simulink model "FlshbcontrolHybridefinal"  (R2020a)
settings: Solver=VariableStepAuto  StartTime=0.0  StopTime=400  RelTol=1e-3
values from neighbouring files (symbols this model uses):
  Acure = Afb    [Initiate.m]
  Afb = [1.9325, 1 ... (first row only)    [Initiate.m]
  Anf = 0.9855    [Initiate.m]
  Anom = 0.9989    [Initiate.m]
  Bcure = 2/7*Bfb    [Initiate.m]
  Bfb = [16.4988 ... (first row only)    [Initiate.m]
  Bnf = -1.5360/4    (= -0.384)    [Initiate.m]
  Bnom = -1.4118e-05    [Initiate.m]
  Ccure = Cfb    [Initiate.m]
  Cfb = [1, 0]    [Initiate.m]
  Cnf = 1    [Initiate.m]
  Cnom = 1    [Initiate.m]
  Dtmax = 2    [Initiate.m]
  dTulim = 3.8    [Initiate.m]
  eta_switch = 0.05    [Initiate.m]
  F = [107.404393816111,9.22073025292975]    [Initiate.m]
  Re2 = [42000000 42000000 42000000 42000000 42000000 42000000 42000000 42000000 42000000 42000000 42000000 42000000 ... (2604 elements, 1302x2)]    [data.mat]
  TC2 = [50.3264 50.3264 50.3264 50.3264 50.3264 50.4703 50.4703 50.3264 50.4703 50.1825 50.4703 50.4703 ... (43248 elements, 10812x4)]    [data.mat]
  Tref = 55*ones(size(t))    [Initiate.m]
  ts = 1/fs    (= 0.02)    [Initiate.m]
libraries: simulink x4, dspsrcs4 x3
settings Model: Creator=Fedor  LastModifiedBy=Fedor
settings SolverCC: ZeroCrossAlgorithm=Adaptive  AlgebraicLoopSolver=LineSearch
settings DebuggingCC: IgnoredZcDiagnostic=none

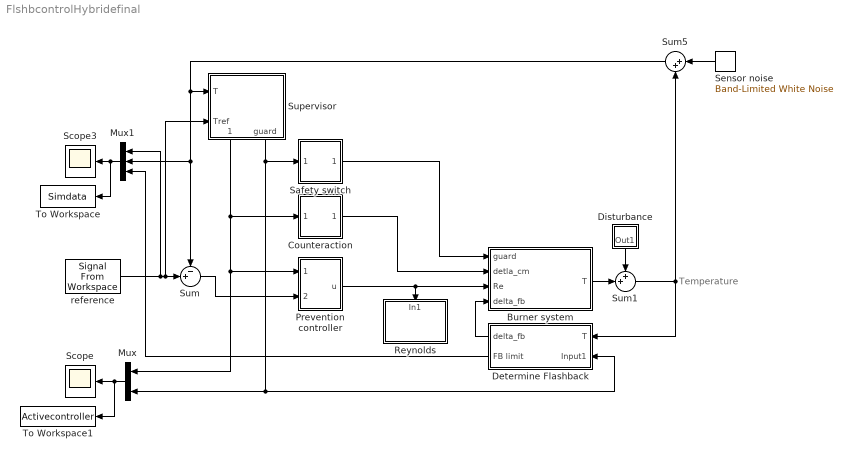
== system FlshbcontrolHybridefinal ==
  note: Temperature
  Burner system : Subsystem
  Counteraction : Subsystem
  Determine Flashback : Subsystem
      settings: PortSchema="{\"entries\":[{\"content\":{\"sides\":[{\"content\":{\"connectorIds\":[\"Out1\",\"Out2\"]},\"type\":\"ConnectorPlacement.EquallySpacedRectSide\",\"uuid\":\"ad351d79-2b46-40dd-a91e-e353291c761f\"},{\"content\":{\"connectorIds\":[\"In1\",\"In2\"],\"side\":\"RIGHT\"},\"type\":\"ConnectorPlacement.EquallySpacedRectSide\",\"uuid\":\"cdcf81d4-3fd0-43bb-8845-11aad52567de\"},{\"content\":{\"connectorIds\":[],\"side\":\"TOP\"},\"type\":\"ConnectorPlacement.EquallySpacedRectSide\",\"uuid\":\"01812f01-e66c-4ed7-90a9-998cda91f1d5\"}]},\"type\":\"ConnectorPlacement.EquallySpacedConnector\",\"uuid\":\"b1549c26-5e6e-49c6-96b0-d801c2fc8257\"}],\"packageUris\":[\"http://schema.mathworks.com/mf0/Connector/19700101\"],\"version\":\"1.0\"}"
  Disturbance : Subsystem
  Mux : Mux  Inputs=2
  Mux1 : Mux  Inputs=3
  Prevention controller : Subsystem
  Reynolds : Subsystem
  Safety switch : Subsystem
  Scope : Scope
  Scope3 : Scope
  Sensor noise : simulink/Sources/Band-Limited White Noise  Cov=[0.01]  Ts=0.1  seed=[23341]
  Sum : Sum  Inputs=-+|
  Sum1 : Sum  Inputs=++|
  Sum5 : Sum  Inputs=|++
  Supervisor : Subsystem
      settings: PortSchema="{\"entries\":[{\"content\":{\"sides\":[{\"content\":{\"connectorIds\":[\"In1\",\"In2\"]},\"type\":\"ConnectorPlacement.EquallySpacedRectSide\",\"uuid\":\"571624c9-6e5f-4ddd-9565-8ab4427e4a42\"},{\"content\":{\"connectorIds\":[],\"side\":\"RIGHT\"},\"type\":\"ConnectorPlacement.EquallySpacedRectSide\",\"uuid\":\"de37e442-dee3-4915-b6ae-6f112b137af7\"},{\"content\":{\"connectorIds\":[],\"side\":\"TOP\"},\"type\":\"ConnectorPlacement.EquallySpacedRectSide\",\"uuid\":\"1a151974-7f5f-47b3-b1fe-80b05a0568b7\"},{\"content\":{\"connectorIds\":[\"Out1\",\"Out2\"],\"side\":\"BOTTOM\"},\"type\":\"ConnectorPlacement.EquallySpacedRectSide\",\"uuid\":\"4bdcf519-e090-41e6-a0b8-d921e146b9ae\"}]},\"type\":\"ConnectorPlacement.EquallySpacedConnector\",\"uuid\":\"70c61ab9-61f6-4665-b82f-34e3b9a13110\"}],\"packageUris\":[\"http://schema.mathworks.com/mf0/Connector/19700101\"],\"version\":\"1.0\"}"
  To Workspace : ToWorkspace  VariableName=Simdata  SampleTime=ts
  To Workspace1 : ToWorkspace  VariableName=Activecontroller  SampleTime=ts
  reference : dspsrcs4/Signal From Workspace  X=Tref  Ts=ts  nsamps=1  OutputAfterFinalValue=Setting to zero  ignoreOrWarnInputAndFrameLengths=off  OutputFrames=off
  wires:
  Mux1/1 -> To Workspace/1, Scope3/1
  Determine Flashback/2(FB limit) -> Mux1/3
  Determine Flashback/1(delta_fb) -> Burner system/4(delta_fb)
  Burner system/1(T) -> Sum1/2
  Prevention controller/1(u) -> Reynolds/1(In1), Burner system/3(Re)
  reference/1 -> Supervisor/2(Tref), Sum/2, Mux1/1
  Sum1/1 -> Sum5/2, Determine Flashback/1(T)
  Sensor noise/1 -> Sum5/1
  Disturbance/1(Out1) -> Sum1/1
  Sum5/1 -> Sum/1, Mux1/2, Supervisor/1(T)
  Supervisor/1(delta_cm) -> Mux/1, Prevention controller/1(Reset), Counteraction/1(Delta_cm)
  Counteraction/1(delta_cm) -> Burner system/2(detla_cm)
  Supervisor/2(guard) -> Safety switch/1(Guard), Determine Flashback/2(Input1), Mux/2
  Mux/1 -> To Workspace1/1, Scope/1
  Sum/1 -> Prevention controller/2(Error)
  Safety switch/1(guard) -> Burner system/1(guard)

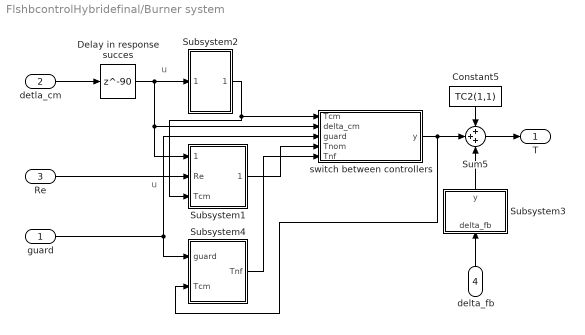
== system FlshbcontrolHybridefinal/Burner system ==
  note: u
  note: u
  guard : Inport
  detla_cm : Inport  Port=2
  Re : Inport  Port=3
  delta_fb : Inport  Port=4
  Constant5 : Constant  Value=TC2(1,1)  SampleTime=ts
  Delay in response succes : Delay  DelayLength=90  SampleTime=ts
  Subsystem1 : Subsystem
  Subsystem2 : Subsystem
  Subsystem3 : Subsystem
  Subsystem4 : Subsystem
  Sum5 : Sum  Inputs=+++
  switch between controllers : MATLAB Function  TreatAsAtomicUnit=on
  T : Outport
  wires:
  Constant5/1 -> Sum5/1
  Sum5/1 -> T/1
  Re/1 -> Subsystem1/2(Re)
  detla_cm/1 -> Delay in response succes/1
  Subsystem1/1(Tnom) -> switch between controllers/4(Tnom)
  Subsystem2/1(Tcm) -> Subsystem1/3(Tcm), switch between controllers/1(Tcm)
  delta_fb/1 -> Subsystem3/1(delta_fb)
  Subsystem3/1(y) -> Sum5/3
  switch between controllers/1(y) -> Subsystem4/2(Tcm), Sum5/2
  guard/1 -> switch between controllers/3(guard), Subsystem4/1(guard)
  Subsystem4/1(Tnf) -> switch between controllers/5(Tnf)
  Delay in response succes/1 -> Subsystem1/1(delta_cm), switch between controllers/2(delta_cm), Subsystem2/1(In1)

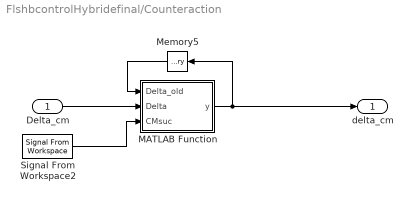
== system FlshbcontrolHybridefinal/Counteraction ==
  Delta_cm : Inport
  MATLAB Function : MATLAB Function  TreatAsAtomicUnit=on
  Memory5 : Memory
  Signal From Workspace2 : dspsrcs4/Signal From Workspace  X=CMsucces  Ts=ts  nsamps=1  OutputAfterFinalValue=Setting to zero  ignoreOrWarnInputAndFrameLengths=off  OutputFrames=off
  delta_cm : Outport
  wires:
  MATLAB Function/1(y) -> delta_cm/1, Memory5/1
  Delta_cm/1 -> MATLAB Function/2(Delta)
  Signal From Workspace2/1 -> MATLAB Function/3(CMsuc)
  Memory5/1 -> MATLAB Function/1(Delta_old)

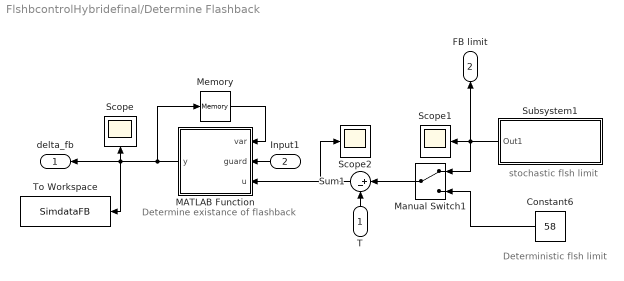
== system FlshbcontrolHybridefinal/Determine Flashback ==
  note: stochastic flsh limit
  note: Deterministic flsh limit
  note: Determine existance of flashback
  T : Inport
  Input1 : Inport  Port=2
  Constant6 : Constant  Value=58
  MATLAB Function : MATLAB Function  TreatAsAtomicUnit=on
  Manual Switch1 : ManualSwitch  Tag=sw1
  Memory : Memory
  Scope : Scope
  Scope1 : Scope
  Scope2 : Scope
  Subsystem1 : Subsystem
  Sum1 : Sum  Inputs=|+-
  To Workspace : ToWorkspace  VariableName=SimdataFB  SampleTime=ts
  delta_fb : Outport
  FB limit : Outport  Port=2
  wires:
  Manual Switch1/1 -> Sum1/1
  Sum1/1 -> Scope2/1, MATLAB Function/3(u)
  MATLAB Function/1(y) -> delta_fb/1, Scope/1, To Workspace/1, Memory/1
  Subsystem1/1(Out1) -> FB limit/1, Scope1/1, Manual Switch1/1
  Constant6/1 -> Manual Switch1/2
  Memory/1 -> MATLAB Function/1(var)
  T/1 -> Sum1/2
  Input1/1 -> MATLAB Function/2(guard)

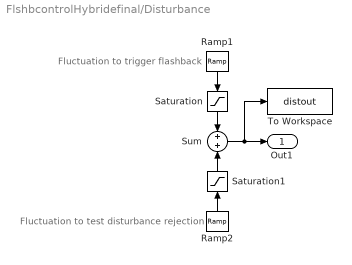
== system FlshbcontrolHybridefinal/Disturbance ==
  note: Fluctuation to trigger flashback
  note: Fluctuation to test disturbance rejection
  Ramp1 : simulink/Sources/Ramp  slope=0  start=200  InitialOutput=0
  Ramp2 : simulink/Sources/Ramp  slope=1  start=100  InitialOutput=0
  Saturation : Saturate  UpperLimit=10  LowerLimit=0
  Saturation1 : Saturate  UpperLimit=5  LowerLimit=0
  Sum : Sum
  To Workspace : ToWorkspace  VariableName=distout  SampleTime=ts
  Out1 : Outport
  wires:
  Ramp1/1 -> Saturation/1
  Sum/1 -> To Workspace/1, Out1/1
  Saturation/1 -> Sum/1
  Saturation1/1 -> Sum/2
  Ramp2/1 -> Saturation1/1

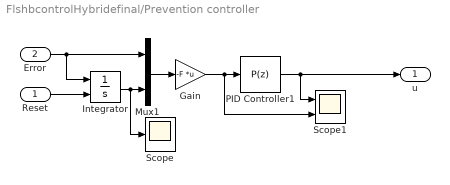
== system FlshbcontrolHybridefinal/Prevention controller ==
  Reset : Inport
  Error : Inport  Port=2
  Gain : Gain  Gain=-F  Multiplication=Matrix(K*u)
  Integrator : Integrator  ExternalReset=falling
  Mux1 : Mux  Inputs=2
  PID Controller1 : simulink/Continuous/PID Controller  Controller=P  Form=Parallel  TimeDomain=Discrete-time  UseExternalTs=off  SampleTime=ts  IntegratorMethod=Forward Euler  FilterMethod=Forward Euler  ControllerParametersSource=internal  P=1  I=F(2)  D=0  UseFilter=on  N=100  TunerSelectOption=Transfer Function Based (PID Tuner App)  InitialConditionSource=internal  InitialConditionForIntegrator=0  InitialConditionForFilter=0  DifferentiatorICPrevScaledInput=0  ExternalReset=falling  TrackingMode=off  Kt=1  LimitOutput=on  UpperSaturationLimit=5000-Re2(1,1)/10000  LowerSaturationLimit=2000-Re2(1,1)/10000  LinearizeAsGain=on  AntiWindupMode=clamping  Kb=1  POutMin=[]  POutMax=[]  IOutMin=[]  IOutMax=[]  DOutMin=[]  DOutMax=[]  NOutMin=[]  NOutMax=[]  SumOutMin=[]  SumOutMax=[]  SaturationOutMin=[]  SaturationOutMax=[]  PParamMin=[]  PParamMax=[]  IParamMin=[]  IParamMax=[]  DParamMin=[]  DParamMax=[]  NParamMin=[]  NParamMax=[]  KbParamMin=[]  KbParamMax=[]  KtParamMin=[]  KtParamMax=[]  KbOutMin=[]  KbOutMax=[]  KtOutMin=[]  KtOutMax=[]  IntegratorOutMin=[]  IntegratorOutMax=[]  FilterOutMin=[]  FilterOutMax=[]  SumI1OutMin=[]  SumI1OutMax=[]  SumI2OutMin=[]  SumI2OutMax=[]  SumI3OutMin=[]  SumI3OutMax=[]  SumI4OutMin=[]  SumI4OutMax=[]  SumDOutMin=[]  SumDOutMax=[]  DifferentiatorOutMin=[]  DifferentiatorOutMax=[]  FilterDiffOutCoefMin=[]  FilterDiffOutCoefMax=[]  ReciprocalOutMin=[]  ReciprocalOutMax=[]  SumDenOutMin=[]  SumDenOutMax=[]  SumNumOutMin=[]  SumNumOutMax=[]  DivideOutMin=[]  DivideOutMax=[]  UdiffTsProdOutMin=[]  UdiffTsProdOutMax=[]  NTsProdOutMin=[]  NTsProdOutMax=[]  UintegralTsProdOutMin=[]  UintegralTsProdOutMax=[]  UngainTsProdOutMin=[]  UngainTsProdOutMax=[]  IntegratorContinuousStateAttributes=''  IntegratorStateMustResolveToSignalObject=off  IntegratorRTWStateStorageClass=Auto  FilterContinuousStateAttributes=''  FilterStateMustResolveToSignalObject=off  FilterRTWStateStorageClass=Auto  ParallelPVariant=InternalParameters  IdealPVariant=Disabled  IVariant=Disabled  DVariant=Disabled  IntegratorVariant=Disabled  SatVariant=Enabled  AWVariant=Disabled  PCopyVariant=Disabled  TRVariant=Disabled  FdbkBlocksVariant=Forward  IdealPFdbkVariant=Disabled  SatFdbkVariant=Disabled  DerivativeFilterVariant=Disabled  NVariant=Disabled  NCopyVariant=Disabled_SignalSpec  FilterICVariant=Disabled  IntegratorICVariant=Disabled  ExternalResetVariant=Disabled  TRSumVariant=Passthrough  SumFdbkVariant=Disabled  SumVariant=Passthrough_P  TsampFilterVariant=InternalTs  TsampNgainVariant=Passthrough  TsampIntegralVariant=Disabled_SignalSpec
  Scope : Scope
  Scope1 : Scope  NumInputPorts=2
  u : Outport
  wires:
  Mux1/1 -> Gain/1
  Integrator/1 -> Scope/1, Mux1/2
  Error/1 -> Mux1/1, Integrator/1
  Reset/1 -> Integrator/2
  Gain/1 -> Scope1/2, PID Controller1/1
  PID Controller1/1 -> u/1, Scope1/1

== system FlshbcontrolHybridefinal/Reynolds ==
  note: Reynolds
  In1 : Inport
  Constant3 : Constant  Value=Re2(1,1)/10000
  Scope4 : Scope
  Sum6 : Sum  Inputs=++|
  To Workspace1 : ToWorkspace  VariableName=SimdataRe  SampleTime=ts
  wires:
  Sum6/1 -> To Workspace1/1, Scope4/1
  Constant3/1 -> Sum6/2
  In1/1 -> Sum6/1

== system FlshbcontrolHybridefinal/Safety switch ==
  Guard : Inport
  guard : Outport
  wires:
  Guard/1 -> guard/1

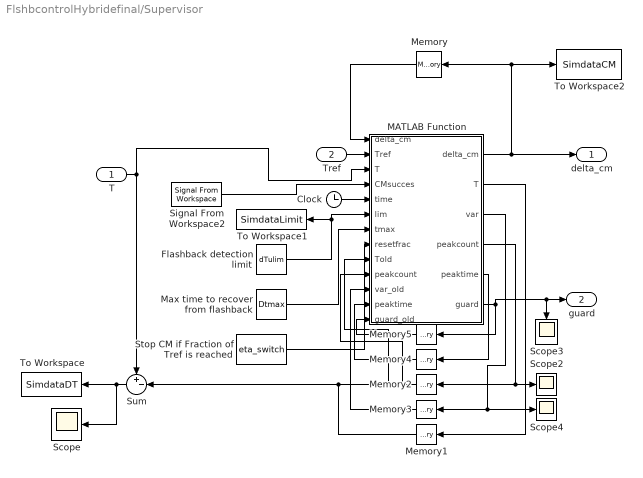
== system FlshbcontrolHybridefinal/Supervisor ==
  T : Inport
  Tref : Inport  Port=2
  Clock : Clock
  Flashback detection limit : Constant  Value=dTulim  SampleTime=ts
  MATLAB Function : MATLAB Function  TreatAsAtomicUnit=on
  Max time to recover from flashback : Constant  Value=Dtmax
  Memory{,2..5} (5 alike) : Memory
  Memory1 : Memory  InitialCondition=Tref(1,1)
  Scope{,2..4} (4 alike) : Scope
  Signal From Workspace2 : dspsrcs4/Signal From Workspace  X=CMsucces  Ts=ts  nsamps=1  OutputAfterFinalValue=Setting to zero  ignoreOrWarnInputAndFrameLengths=off  OutputFrames=off
  Stop CM if Fraction of Tref is reached : Constant  Value=eta_switch
  Sum : Sum  Inputs=+-|
  To Workspace : ToWorkspace  VariableName=SimdataDT  SampleTime=ts
  To Workspace1 : ToWorkspace  VariableName=SimdataLimit  SampleTime=ts
  To Workspace2 : ToWorkspace  VariableName=SimdataCM  SampleTime=ts
  delta_cm : Outport
  guard : Outport  Port=2
  wires:
  Clock/1 -> MATLAB Function/5(time)
  Flashback detection limit/1 -> MATLAB Function/6(lim), To Workspace1/1
  Memory/1 -> MATLAB Function/1("delta_cm ")
  MATLAB Function/2(T) -> Memory1/1
  MATLAB Function/1(delta_cm) -> To Workspace2/1, Memory/1, delta_cm/1
  Memory1/1 -> MATLAB Function/9(Told), Sum/2
  Sum/1 -> To Workspace/1, Scope/1
  MATLAB Function/4(peakcount) -> Memory2/1, Scope2/1
  Memory2/1 -> MATLAB Function/10("peakcount ")
  MATLAB Function/3(var) -> Memory3/1, Scope4/1
  Memory3/1 -> MATLAB Function/11(var_old)
  T/1 -> Sum/1, MATLAB Function/3("T ")
  Signal From Workspace2/1 -> MATLAB Function/4(CMsucces)
  MATLAB Function/5(peaktime) -> Memory4/1
  Memory4/1 -> MATLAB Function/12("peaktime ")
  MATLAB Function/6(guard) -> guard/1, Scope3/1, Memory5/1
  Tref/1 -> MATLAB Function/2(Tref)
  Memory5/1 -> MATLAB Function/13(guard_old)
  Max time to recover from flashback/1 -> MATLAB Function/7(tmax)
  Stop CM if Fraction of Tref is reached/1 -> MATLAB Function/8(resetfrac)

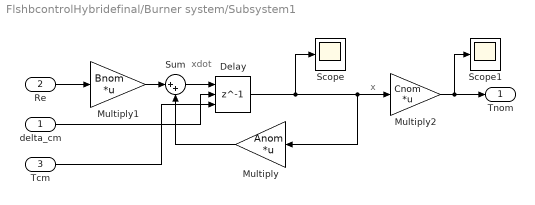
== system FlshbcontrolHybridefinal/Burner system/Subsystem1 ==
  note: x
  note: xdot
  delta_cm : Inport
  Re : Inport  Port=2
  Tcm : Inport  Port=3
  Delay : Delay  DelayLength=1  InitialConditionSource=Input port  ExternalReset=Falling  SampleTime=ts
      settings: InputPortMap=u0,r5,p4
  Multiply : Gain  Gain=Anom  Multiplication=Matrix(K*u)
  Multiply1 : Gain  Gain=Bnom  Multiplication=Matrix(K*u)
  Multiply2 : Gain  Gain=Cnom  Multiplication=Matrix(K*u)
  Scope : Scope
  Scope1 : Scope
  Sum : Sum  Inputs=|++
  Tnom : Outport
  wires:
  Multiply2/1 -> Scope1/1, Tnom/1
  Sum/1 -> Delay/1
  Delay/1 -> Scope/1, Multiply2/1, Multiply/1
  Multiply1/1 -> Sum/1
  Multiply/1 -> Sum/2
  Re/1 -> Multiply1/1
  Tcm/1 -> Delay/3
  delta_cm/1 -> Delay/2

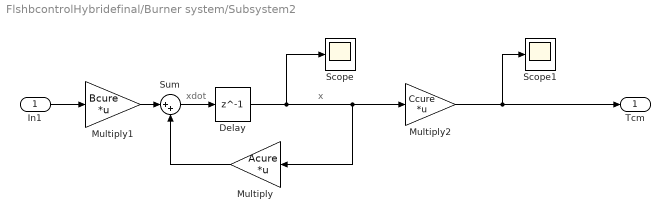
== system FlshbcontrolHybridefinal/Burner system/Subsystem2 ==
  note: x
  note: xdot
  In1 : Inport
  Delay : Delay  DelayLength=1  SampleTime=ts
  Multiply : Gain  Gain=Acure  Multiplication=Matrix(K*u)
  Multiply1 : Gain  Gain=Bcure  Multiplication=Matrix(K*u)
  Multiply2 : Gain  Gain=Ccure  Multiplication=Matrix(K*u)
  Scope : Scope
  Scope1 : Scope
  Sum : Sum  Inputs=|++
  Tcm : Outport
  wires:
  Multiply2/1 -> Scope1/1, Tcm/1
  Sum/1 -> Delay/1
  Delay/1 -> Scope/1, Multiply/1, Multiply2/1
  Multiply1/1 -> Sum/1
  Multiply/1 -> Sum/2
  In1/1 -> Multiply1/1

== system FlshbcontrolHybridefinal/Burner system/Subsystem3 ==
  delta_fb : Inport
  MATLAB Function1 : MATLAB Function  TreatAsAtomicUnit=on
  Memory : Memory
  Subsystem : Subsystem
  y : Outport
  wires:
  delta_fb/1 -> Subsystem/1(In1), MATLAB Function1/2(delta_fb)
  Subsystem/1(Tnom) -> MATLAB Function1/1(Tcm)
  MATLAB Function1/1(y) -> y/1
  MATLAB Function1/2(beta) -> Memory/1
  Memory/1 -> MATLAB Function1/3("beta ")

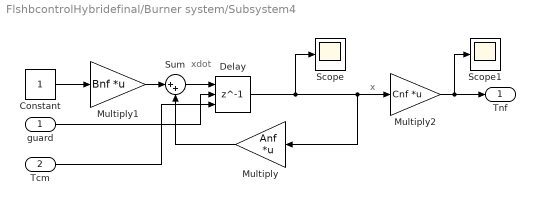
== system FlshbcontrolHybridefinal/Burner system/Subsystem4 ==
  note: x
  note: xdot
  guard : Inport
  Tcm : Inport  Port=2
  Constant : Constant
  Delay : Delay  DelayLength=1  InitialConditionSource=Input port  ShowEnablePort=on  SampleTime=ts
      settings: InputPortMap=u0,e6,p4
  Multiply : Gain  Gain=Anf  Multiplication=Matrix(K*u)
  Multiply1 : Gain  Gain=Bnf  Multiplication=Matrix(K*u)
  Multiply2 : Gain  Gain=Cnf  Multiplication=Matrix(K*u)
  Scope : Scope
  Scope1 : Scope
  Sum : Sum  Inputs=|++
  Tnf : Outport
  wires:
  Multiply2/1 -> Scope1/1, Tnf/1
  Sum/1 -> Delay/1
  Delay/1 -> Scope/1, Multiply2/1, Multiply/1
  Multiply1/1 -> Sum/1
  Multiply/1 -> Sum/2
  Tcm/1 -> Delay/3
  guard/1 -> Delay/2
  Constant/1 -> Multiply1/1

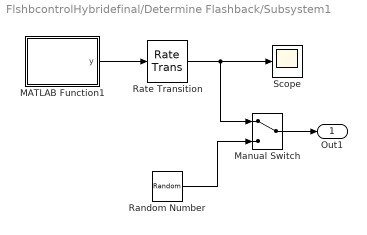
== system FlshbcontrolHybridefinal/Determine Flashback/Subsystem1 ==
  MATLAB Function1 : MATLAB Function  TreatAsAtomicUnit=on
  Manual Switch : ManualSwitch
  Random Number : RandomNumber  Mean=71.1  Variance=3.7  SampleTime=2
  Rate Transition : RateTransition  OutPortSampleTime=1
  Scope : Scope
  Out1 : Outport
  wires:
  Manual Switch/1 -> Out1/1
  Random Number/1 -> Manual Switch/2
  MATLAB Function1/1(y) -> Rate Transition/1
  Rate Transition/1 -> Scope/1, Manual Switch/1

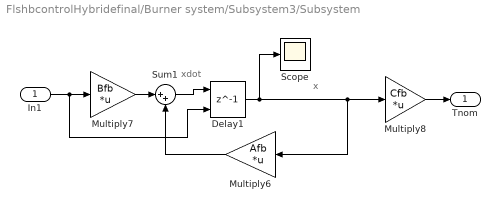
== system FlshbcontrolHybridefinal/Burner system/Subsystem3/Subsystem ==
  note: x
  note: xdot
  In1 : Inport
  Delay1 : Delay  DelayLength=1  ExternalReset=Falling  SampleTime=ts
      settings: InputPortMap=u0,r5
  Multiply6 : Gain  Gain=Afb  Multiplication=Matrix(K*u)
  Multiply7 : Gain  Gain=Bfb  Multiplication=Matrix(K*u)
  Multiply8 : Gain  Gain=Cfb  Multiplication=Matrix(K*u)
  Scope : Scope
  Sum1 : Sum  Inputs=|++
  Tnom : Outport
  wires:
  Sum1/1 -> Delay1/1
  Delay1/1 -> Scope/1, Multiply8/1, Multiply6/1
  Multiply8/1 -> Tnom/1
  In1/1 -> Delay1/2, Multiply7/1
  Multiply7/1 -> Sum1/1
  Multiply6/1 -> Sum1/2

== matlab function FlshbcontrolHybridefinal/Counteraction/MATLAB Function ==
  data: Delta_old input; Delta input; y output; CMsuc input
function y = fcn(Delta_old, Delta, CMsuc)
if CMsuc < 1 && Delta == 1
    y = Delta_old;
else
    y = Delta;
end

== matlab function FlshbcontrolHybridefinal/Burner system/switch between controllers ==
  data: Tcm input; delta_cm input; guard input; Tnom input; y output; Tnf input
function y = switching(Tcm, delta_cm, guard, Tnom, Tnf)
if guard == 1
    y = Tnf;
elseif delta_cm > 0 && guard == 0
    y = Tcm;    
else
    y = Tnom;
end
end

== matlab function FlshbcontrolHybridefinal/Determine Flashback/MATLAB Function ==
  data: var input; guard input; u input; y output
function y = flashback(var, guard, u)

    if u<0
        var = 1;
    elseif u>= 0 && guard ==0
        var = 0;
    end
    
    y = var;
end

== matlab function FlshbcontrolHybridefinal/Burner system/Subsystem3/MATLAB Function1 ==
  data: Tcm input; delta_fb input; y output; beta output; beta input
function [y,beta] = fcn(Tcm, delta_fb, beta)

if delta_fb > 0
    y = Tcm;
    beta = Tcm;
else 
    y = beta*0.9;
    beta = 0.9*beta;
end

== matlab function FlshbcontrolHybridefinal/Determine Flashback/Subsystem1/MATLAB Function1 ==
  data: y output
function y = uniform()
a = 61;
b = 70;
% a = 71;
% b = 80;
y = a + rand(1)*(b-a);

== matlab function FlshbcontrolHybridefinal/Supervisor/MATLAB Function ==
  data: delta_cm input; Tref input; T input; CMsucces input; time input; lim input; tmax input; resetfrac input; Told input; peakcount input; var_old input; delta_cm output; T output; var output; peakcount output; peaktime output; peaktime input; guard output; guard_old input
function [delta_cm,T, var,peakcount, peaktime, guard] = supervisor(delta_cm,Tref,  T, CMsucces, time, lim, tmax, resetfrac, Told,peakcount, var_old, peaktime, guard_old)
    % Compare current temperature to old temperature if it exceeds the FB
    % limit
    if (T-Told)>lim
        var = 1;
    else
        var = 0;
    end
    
    % Check if there is peak detected and if yes increase the peak counter
    if var-var_old > 0 
       peakcount = peakcount + 1;
       peaktime = time;
    end
    
    % If this is the first time step, where peak is uneven again, activate
    % counter measure and deactivate if temperature is back within 10% ref or
    % counter measure has failed
    if mod(peakcount,2)==1 && var-var_old > 0 %&& CMsucces==1
        delta_cm = 1;
    elseif (T-Tref)/Tref < resetfrac && guard_old == 0
        delta_cm = 0;
    elseif guard_old == 1
        delta_cm = 0;
    end
    
    % Activate guard if takes more than 2 seconds before second peak
    % detection
    if mod(peakcount,2)==1 && time - peaktime > tmax
        guard = 1;
    else
        guard = guard_old;
    end
    
end
